simulink model "SimulationLQR_NaoLinear"  (R2024b)
settings: Solver=VariableStepAuto  StartTime=0.0  StopTime=10  MaxStep=0.01  RelTol=1e-10
undefined symbols (not defined in the file): K
settings Model: Creator=Igor  LastModifiedBy=ybern

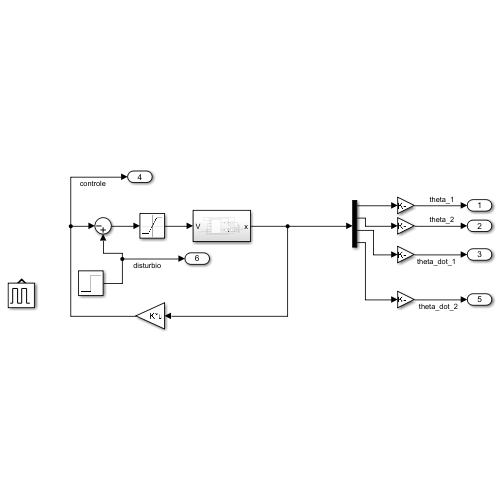
[thumbnail: Simulink's stored preview of the top-level diagram]
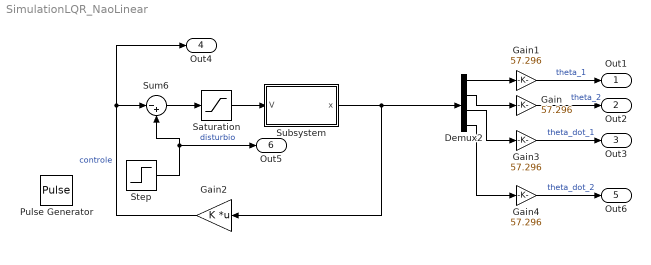
== system SimulationLQR_NaoLinear ==
  Demux2 : Demux
  Gain{,1,3..4} (4 alike) : Gain  Gain=57.296
  Gain2 : Gain  Gain=K  Multiplication=Matrix(K*u)
  Pulse Generator : DiscretePulseGenerator  PulseType=Time based  Period=10  PulseWidth=10
  Saturation : Saturate  UpperLimit=12  LowerLimit=-12
  Step : Step  SampleTime=0
  Subsystem : Subsystem
  Sum6 : Sum  Inputs=|-+
  Out1 : Outport
  Out2 : Outport  Port=2
  Out3 : Outport  Port=3
  Out4 : Outport  Port=4
  Out6 : Outport  Port=5
  Out5 : Outport  Port=6
  wires:
  Demux2/3 -> Gain3/1
  Sum6/1 -> Saturation/1
  Gain2/1 -> Sum6/1, Out4/1  "controle"
  Demux2/1 -> Gain1/1
  Demux2/2 -> Gain/1
  Gain/1 -> Out2/1  "theta_2"
  Gain1/1 -> Out1/1  "theta_1"
  Demux2/4 -> Gain4/1
  Gain3/1 -> Out3/1  "theta_dot_1"
  Gain4/1 -> Out6/1  "theta_dot_2"
  Subsystem/1(x) -> Gain2/1, Demux2/1
  Saturation/1 -> Subsystem/1(V)
  Step/1 -> Out5/1, Sum6/2  "disturbio"

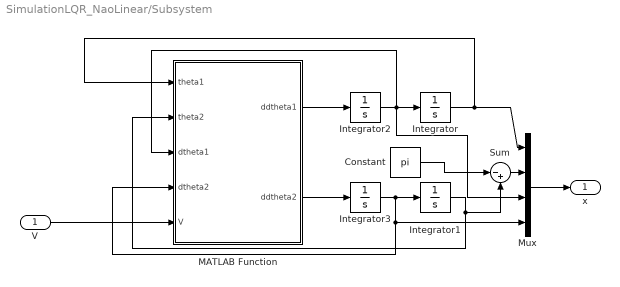
== system SimulationLQR_NaoLinear/Subsystem ==
  V : Inport
  Constant : Constant  Value=pi
  Integrator : Integrator
  Integrator1 : Integrator  InitialCondition=pi
  Integrator2 : Integrator
  Integrator3 : Integrator
  MATLAB Function : MATLAB Function  TreatAsAtomicUnit=on
  Mux : Mux
  Sum : Sum  Inputs=|-+
  x : Outport
  wires:
  MATLAB Function/1(ddtheta1) -> Integrator2/1
  MATLAB Function/2(ddtheta2) -> Integrator3/1
  Integrator2/1 -> Mux/3, MATLAB Function/3(dtheta1), Integrator/1
  Integrator3/1 -> MATLAB Function/4(dtheta2), Mux/4, Integrator1/1
  Integrator1/1 -> Sum/2, MATLAB Function/2(theta2)
  Integrator/1 -> Mux/1, MATLAB Function/1(theta1)
  Mux/1 -> x/1
  V/1 -> MATLAB Function/5(V)
  Sum/1 -> Mux/2
  Constant/1 -> Sum/1

== matlab function SimulationLQR_NaoLinear/Subsystem/MATLAB Function ==
  data: theta1 input; theta2 input; dtheta1 input; ddtheta1 output; dtheta2 input; V input; ddtheta2 output
function [ddtheta1, ddtheta2] = furuta_dynamics(theta1, theta2, dtheta1, dtheta2, V)

% Declaração das constantes
g = 9.8; 
J0_hat = 86.27e-6; 
J2_hat = 96.35e-6; 
m2 = 0.016; 
L1 = 0.0362; 
L2 = 0.10;
l1 = 0.028;
l2 = 0.073; 
b1 = 1.33e-4; 
b2 = 2.8e-4;
c1 = 106.99; 
c2 = 5.61; 

% 1. CÁLCULO DOS TORQUES DE ENTRADA
tau1 = J0_hat * (c1 * V - c2 * dtheta1);
tau2 = 0;

% 2. CÁLCULO DAS ACELERAÇÕES (Equações de Furuta)

% Denominador (D)
D = (J0_hat * J2_hat + J2_hat^2 * sin(theta2)^2 - m2^2 * L1^2 * l2^2 * cos(theta2)^2);

% Numerador de ddot_theta1 (Num1)
Num1_term1 = [-J2_hat*b1; m2*L1*l2*cos(theta2)*b2; -J2_hat^2*sin(2*theta2); 
              -0.5*J2_hat*m2*L1*l2*cos(theta2)*sin(2*theta2); J2_hat*m2*L1*l2*sin(theta2)]';
Vec1_states = [dtheta1; dtheta2; dtheta1*dtheta2; dtheta1^2; dtheta2^2];

Num1_term2 = [J2_hat; -m2*L1*l2*cos(theta2); 0.5*m2^2*l2^2*L1*sin(2*theta2)]';
Vec1_inputs = [tau1; tau2; g];

Num1 = Num1_term1 * Vec1_states + Num1_term2 * Vec1_inputs;
ddtheta1 = Num1 / D;

% Numerador de ddot_theta2 (Num2)
Num2_term1 = [m2*L1*l2*cos(theta2)*b1; -b2*(J0_hat + J2_hat*sin(theta2)^2); 
              m2*L1*l2*J2_hat*cos(theta2)*sin(2*theta2); 
              -0.5*sin(2*theta2)*(J0_hat * J2_hat + J2_hat^2 * sin(theta2)^2); 
              -0.5*m2^2*L1^2*l2^2*sin(2*theta2)]';
Vec2_states = [dtheta1; dtheta2; dtheta1*dtheta2; dtheta1^2; dtheta2^2];

Num2_term2 = [-m2*L1*l2*cos(theta2); J0_hat + J2_hat*sin(theta2)^2; 
              -m2*l2*sin(theta2)*(J0_hat + J2_hat*sin(theta2)^2)]';
Vec2_inputs = [tau1; tau2; g];

Num2 = Num2_term1 * Vec2_states + Num2_term2 * Vec2_inputs;
ddtheta2 = Num2 / D;

end
